simulink model "Scattering_based_Position_Position_discrete"  (R2020b)
settings: Solver=VariableStepAuto  StartTime=0.0  StopTime=10  RelTol=1e-3
values from neighbouring files (symbols this model uses):
  Amp = 1    [parameters_Position_Position.m]    (also in parameters_Position_Position_kalman.m)
  b = 1    [parameters_Position_Position.m]    (also in parameters_Position_Position_kalman.m)
  Be = 10    [parameters_Position_Position.m]    (also in parameters_Position_Position_kalman.m)
  Bh = 1.5    [parameters_Position_Position.m]    (also in parameters_Position_Position_kalman.m)
  Bm = 100    [parameters_Position_Position.m]    (also in parameters_Position_Position_kalman.m)
  Bs = 100    [parameters_Position_Position.m]    (also in parameters_Position_Position_kalman.m)
  delay = 1    [parameters_Position_Position.m]    (also in parameters_Position_Position_kalman.m)
  Dm = 0    [parameters_Position_Position.m]    (also in parameters_Position_Position_kalman.m)
  Ds = 0    [parameters_Position_Position.m]    (also in parameters_Position_Position_kalman.m)
  Fc = 0.5    [parameters_Position_Position.m]    (also in parameters_Position_Position_kalman.m)
  Fip = 100    [parameters_Position_Position.m]    (also in parameters_Position_Position_kalman.m)
  Ih = 5    [parameters_Position_Position.m]    (also in parameters_Position_Position_kalman.m)
  Je = 0    [parameters_Position_Position.m]    (also in parameters_Position_Position_kalman.m)
  Jh = 0    [parameters_Position_Position.m]    (also in parameters_Position_Position_kalman.m)
  Ke = 10    [parameters_Position_Position.m]    (also in parameters_Position_Position_kalman.m)
  Kh = 1    [parameters_Position_Position.m]    (also in parameters_Position_Position_kalman.m)
  Km = 50    [parameters_Position_Position.m]    (also in parameters_Position_Position_kalman.m)
  Ks = 80    [parameters_Position_Position.m]    (also in parameters_Position_Position_kalman.m)
  Mm = 0.5    [parameters_Position_Position.m]    (also in parameters_Position_Position_kalman.m)
  Ms = 2    [parameters_Position_Position.m]    (also in parameters_Position_Position_kalman.m)
  Ph = 5    [parameters_Position_Position.m]    (also in parameters_Position_Position_kalman.m)
  tau = 100000    [parameters_Position_Position.m]    (also in parameters_Position_Position_kalman.m)
  Ts = 0.001    [parameters_Position_Position.m]    (also in parameters_Position_Position_kalman.m)
undefined symbols (not defined in the file or in its folder): DiscIntNeverNeededParam
libraries: simulink x2
settings Model: Creator=anuj  LastModifiedBy=Edoardo

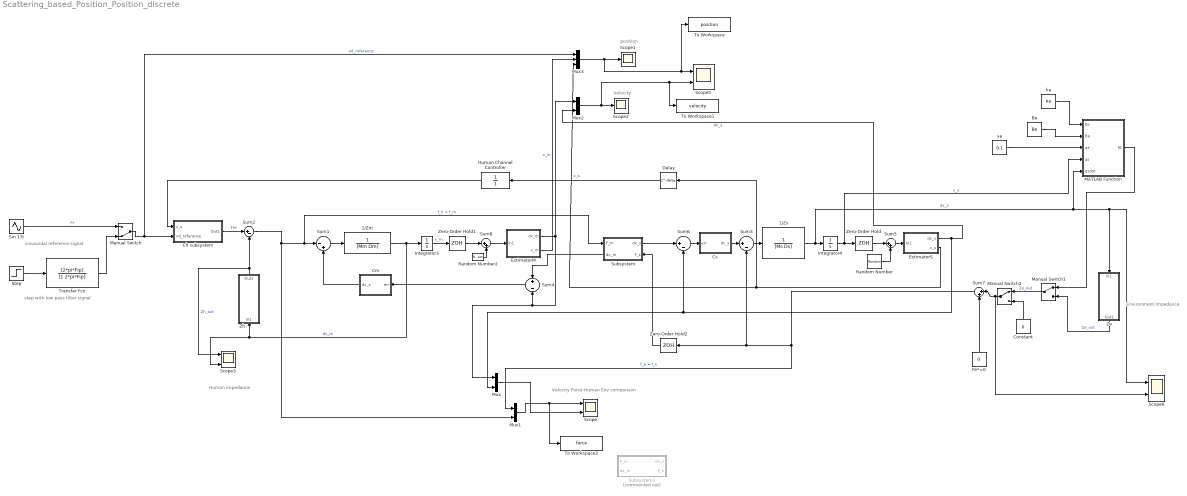
== system Scattering_based_Position_Position_discrete ==
  note: Velocity
  note: position
  note: Environment Impedance
  note: Human impedance
  note: Velocity Force Human Env comparison
  note: sinusoidal reference signal
  note: step with low pass filter signal
  1/Zm : TransferFcn  Denominator=[Mm Dm]
  1/Zs : TransferFcn  Denominator=[Ms Ds]
  Be : Constant  Value=Be
  Ch subsystem : Subsystem
  Cm : Subsystem
  Constant : Constant  Value=0
  Cs : Subsystem
  Delay : Delay  DelayLength=delay  SampleTime=Ts
  EstimatorM : Subsystem
  EstimatorS : Subsystem
  Fe*=0 : Constant  Value=0
  Human Channel Controller : TransferFcn  Denominator=[1]
  Integrator3 : Integrator
  Integrator4 : Integrator
  MATLAB Function : MATLAB Function  TreatAsAtomicUnit=on
  Manual Switch : ManualSwitch  CurrentSetting=0
  Manual Switch1 : ManualSwitch
  Manual Switch2 : ManualSwitch
  Mux : Mux  Inputs=2
  Mux1 : Mux  Inputs=2
  Mux2 : Mux  Inputs=2
  Mux3 : Mux  Inputs=3
  Random Number : RandomNumber  Variance=0  SampleTime=0.1
  Random Number2 : RandomNumber  Variance=0  SampleTime=0.1
  Scope{,3,5..6} (4 alike) : Scope  NumInputPorts=2
  Scope1 : Scope
  Scope2 : Scope
  Sin 17t : Sin  Amplitude=Amp  Frequency=2*pi*Fc  SampleTime=0
  Step : Step  After=Amp  SampleTime=0
  Subsystem : Subsystem
      settings: PortSchema="{\"entries\":[{\"content\":{\"sides\":[{\"content\":{\"connectorIds\":[\"In1\",\"Out2\"]},\"type\":\"ConnectorPlacement.EquallySpacedRectSide\",\"uuid\":\"a4d8a1e6-493d-445f-9b62-4880423e0f65\"},{\"content\":{\"connectorIds\":[\"Out1\",\"In2\"],\"side\":\"RIGHT\"},\"type\":\"ConnectorPlacement.EquallySpacedRectSide\",\"uuid\":\"3d032ce1-a127-47bd-8907-4bd2e1f875d6\"},{\"content\":{\"connectorIds\":[],\"side\":\"TOP\"},\"type\":\"ConnectorPlacement.EquallySpacedRectSide\",\"uuid\":\"51a1971f-6e89-4837-8aa9-c8a237b527d1\"},{\"content\":{\"connectorIds\":[],\"side\":\"HIDDEN\"},\"type\":\"ConnectorPlacement.EquallySpacedRectSide\",\"uuid\":\"2bd12734-fa67-440d-bc97-b4fe58bfa138\"}]},\"type\":\"ConnectorPlacement.EquallySpacedConnector\",\"uuid\":\"cc0f3456-b5e1-4f18-b500-07b4336c0d17\"}],\"packageUris\":[\"http://schema.mathworks.com/mf0/Connector/R2020b\"],\"version\":\"1.0\"}"
  Subsystem1 : Subsystem  Commented=on
      settings: PortSchema="{\"entries\":[{\"content\":{\"sides\":[{\"content\":{\"connectorIds\":[\"In1\",\"Out2\"]},\"type\":\"ConnectorPlacement.EquallySpacedRectSide\",\"uuid\":\"06c9fa59-43a1-4b94-81eb-aaec109dce8e\"},{\"content\":{\"connectorIds\":[\"Out1\",\"In2\"],\"side\":\"RIGHT\"},\"type\":\"ConnectorPlacement.EquallySpacedRectSide\",\"uuid\":\"3f5f1dc1-0465-4088-8d45-d4d0bf9b65eb\"},{\"content\":{\"connectorIds\":[],\"side\":\"TOP\"},\"type\":\"ConnectorPlacement.EquallySpacedRectSide\",\"uuid\":\"9f406951-78e1-44a4-92d9-8338b6137a61\"},{\"content\":{\"connectorIds\":[],\"side\":\"HIDDEN\"},\"type\":\"ConnectorPlacement.EquallySpacedRectSide\",\"uuid\":\"c520c54c-b8c0-41cc-b366-9b185ca7cd6e\"}]},\"type\":\"ConnectorPlacement.EquallySpacedConnector\",\"uuid\":\"d081af34-e020-4561-aa1f-800c2949a30c\"}],\"packageUris\":[\"http://schema.mathworks.com/mf0/Connector/R2020b\"],\"version\":\"1.0\"}"
  Sum1 : Sum  Inputs=|-+
  Sum2 : Sum  Inputs=|+-
  Sum3 : Sum  Inputs=|+-
  Sum4 : Sum  Inputs=+-
  Sum5 : Sum  Inputs=|++
  Sum6 : Sum  Inputs=|+-
  Sum7 : Sum  Inputs=|++
  Sum8 : Sum  Inputs=|++
  To Workspace : ToWorkspace  VariableName=position  SaveFormat=Timeseries  SampleTime=-1
  To Workspace1 : ToWorkspace  VariableName=velocity  SaveFormat=Timeseries  SampleTime=-1
  To Workspace2 : ToWorkspace  VariableName=force  SaveFormat=Timeseries  SampleTime=-1
  Transfer Fcn : TransferFcn  Numerator=[2*pi*Fip]  Denominator=[1 2*pi*Fip]
  Ze : Subsystem
  Zero-Order Hold : ZeroOrderHold  SampleTime=Ts
  Zero-Order Hold1 : ZeroOrderHold  SampleTime=Ts
  Zero-Order Hold2 : ZeroOrderHold  SampleTime=-1
  Zh : Subsystem
  ke : Constant  Value=Ke
  xe : Constant  Value=0.1
  wires:
  Mux/1 -> Scope/2
  Mux1/1 -> Scope/1, To Workspace2/1
  Sum2/1 -> Subsystem/1(F_m), Sum1/1, Mux1/2  "f_h = f_m"
  Sum1/1 -> 1/Zm/1
  Sum3/1 -> 1/Zs/1
  Fe*=0/1 -> Sum7/2
  Sum7/1 -> Mux1/1, Zero-Order Hold2/1, Sum3/2  "f_e = f_s"
  Ch subsystem/1(Out1) -> Sum2/1  "Fh*"
  Be/1 -> MATLAB Function/2(Be)
  xe/1 -> MATLAB Function/3(qe)
  ke/1 -> MATLAB Function/1(Ke)
  Transfer Fcn/1 -> Manual Switch/2
  Step/1 -> Transfer Fcn/1
  Human Channel Controller/1 -> Ch subsystem/1(x_s)
  Manual Switch/1 -> Mux3/1, Ch subsystem/2(xd_reference)  "xd_reference"
  Sin 17t/1 -> Manual Switch/1  "F*"
  MATLAB Function/1(fE) -> Manual Switch1/1
  Manual Switch1/1 -> Manual Switch2/1  "Ze_out"
  Zh/1(Out1) -> Sum2/2, Scope3/1  "Zh_out"
  Ze/1(Out1) -> Manual Switch1/2  "Ze_out"
  Mux2/1 -> Scope2/1, To Workspace1/1, Scope5/2
  Mux3/1 -> Scope1/1, To Workspace/1, Scope5/1
  Sum8/1 -> EstimatorM/1(In1)
  Random Number2/1 -> Sum8/2
  1/Zm/1 -> Integrator3/1, Zh/1(In1), Scope3/2  "dx_m"
  Zero-Order Hold1/1 -> Sum8/1
  Integrator3/1 -> Zero-Order Hold1/1  "x_m"
  EstimatorM/1(dx_m) -> Mux2/1, Sum4/2, Mux/1
  Sum5/1 -> EstimatorS/1(In1)
  Random Number/1 -> Sum5/2
  Zero-Order Hold/1 -> Sum5/1
  Integrator4/1 -> Zero-Order Hold/1, MATLAB Function/4(qs)  "x_s"
  EstimatorS/2(x_s) -> Delay/1, Mux3/3  "x_s"
  EstimatorS/1(dx_s) -> Mux/2, Sum6/2, Mux2/2  "dx_s"
  1/Zs/1 -> Ze/1(In1), Scope6/1, MATLAB Function/5(qsdot), Integrator4/1  "dx_s"
  EstimatorM/2(x_m) -> Mux3/2  "x_m"
  Zero-Order Hold2/1 -> Subsystem/2(F_s)
  Cs/1(dx_s) -> Sum3/1
  Subsystem/1(dx_s) -> Sum6/1
  Sum6/1 -> Cs/1(err)
  Manual Switch2/1 -> Scope6/2, Sum7/1
  Constant/1 -> Manual Switch2/2
  Subsystem/2(dx_m) -> Sum4/1
  Sum4/1 -> Cm/1(err)
  Cm/1(dx_s) -> Sum1/2
  Delay/1 -> Human Channel Controller/1

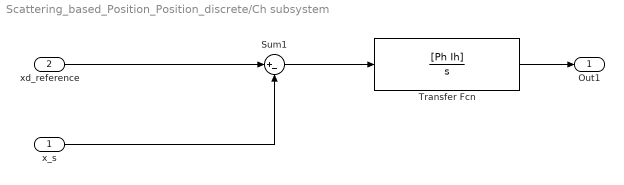
== system Scattering_based_Position_Position_discrete/Ch subsystem ==
  x_s : Inport
  xd_reference : Inport  Port=2
  Sum1 : Sum  Inputs=|+-
  Transfer Fcn : TransferFcn  Numerator=[Ph Ih]  Denominator=[1 0]
  Out1 : Outport
  wires:
  x_s/1 -> Sum1/2
  Sum1/1 -> Transfer Fcn/1
  xd_reference/1 -> Sum1/1
  Transfer Fcn/1 -> Out1/1

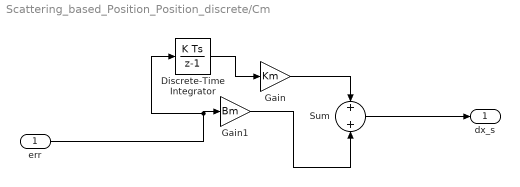
== system Scattering_based_Position_Position_discrete/Cm ==
  err : Inport
  Discrete-Time Integrator : DiscreteIntegrator  SampleTime=Ts  ICPrevOutput=DiscIntNeverNeededParam  ICPrevScaledInput=DiscIntNeverNeededParam
  Gain : Gain  Gain=Km
  Gain1 : Gain  Gain=Bm
  Sum : Sum
  dx_s : Outport
  wires:
  Gain1/1 -> Sum/2
  err/1 -> Discrete-Time Integrator/1, Gain1/1
  Discrete-Time Integrator/1 -> Gain/1
  Gain/1 -> Sum/1
  Sum/1 -> dx_s/1

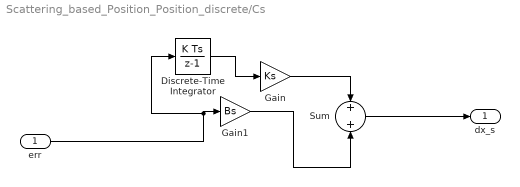
== system Scattering_based_Position_Position_discrete/Cs ==
  err : Inport
  Discrete-Time Integrator : DiscreteIntegrator  SampleTime=Ts  ICPrevOutput=DiscIntNeverNeededParam  ICPrevScaledInput=DiscIntNeverNeededParam
  Gain : Gain  Gain=Ks
  Gain1 : Gain  Gain=Bs
  Sum : Sum
  dx_s : Outport
  wires:
  Gain1/1 -> Sum/2
  err/1 -> Discrete-Time Integrator/1, Gain1/1
  Discrete-Time Integrator/1 -> Gain/1
  Gain/1 -> Sum/1
  Sum/1 -> dx_s/1

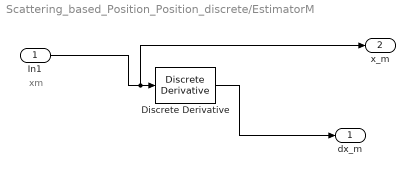
== system Scattering_based_Position_Position_discrete/EstimatorM ==
  note: xm
  In1 : Inport
  Discrete Derivative : simulink/Discrete/Discrete Derivative  gainval=1.0  ICPrevScaledInput=0.0  OutMin=[]  OutMax=[]  OutDataType=fixdt(1, 16)  OutScaling=2^-10  DoSatur=off
  dx_m : Outport
  x_m : Outport  Port=2
  wires:
  Discrete Derivative/1 -> dx_m/1
  In1/1 -> x_m/1, Discrete Derivative/1

== system Scattering_based_Position_Position_discrete/EstimatorS ==
  note: xs
  In1 : Inport
  Discrete Derivative : simulink/Discrete/Discrete Derivative  gainval=1.0  ICPrevScaledInput=0.0  OutMin=[]  OutMax=[]  OutDataType=fixdt(1, 16)  OutScaling=2^-10  DoSatur=off
  dx_s : Outport
  x_s : Outport  Port=2
  wires:
  In1/1 -> x_s/1, Discrete Derivative/1
  Discrete Derivative/1 -> dx_s/1

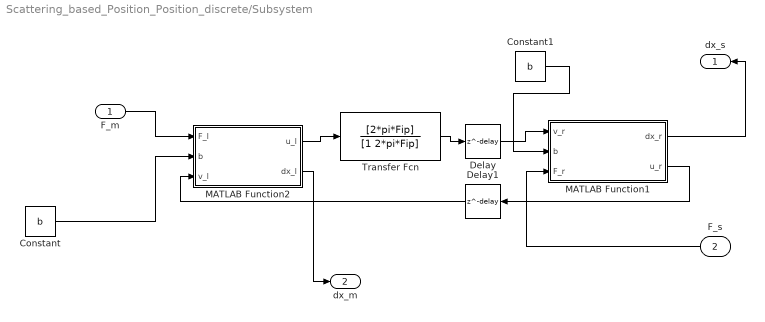
== system Scattering_based_Position_Position_discrete/Subsystem ==
  F_m : Inport
  F_s : Inport  Port=2
  Constant : Constant  Value=b
  Constant1 : Constant  Value=b
  Delay : Delay  DelayLength=delay  SampleTime=Ts
  Delay1 : Delay  DelayLength=delay  SampleTime=Ts
  MATLAB Function1 : MATLAB Function  TreatAsAtomicUnit=on
  MATLAB Function2 : MATLAB Function  TreatAsAtomicUnit=on
  Transfer Fcn : TransferFcn  Numerator=[2*pi*Fip]  Denominator=[1 2*pi*Fip]
  dx_s : Outport
  dx_m : Outport  Port=2
  wires:
  F_m/1 -> MATLAB Function2/1(F_l)
  MATLAB Function2/2(dx_l) -> dx_m/1
  MATLAB Function2/1(u_l) -> Transfer Fcn/1
  Delay/1 -> MATLAB Function1/1(v_r)
  Delay1/1 -> MATLAB Function2/3(v_l)
  MATLAB Function1/2(u_r) -> Delay1/1
  MATLAB Function1/1(dx_r) -> dx_s/1
  F_s/1 -> MATLAB Function1/3(F_r)
  Constant/1 -> MATLAB Function2/2(b)
  Constant1/1 -> MATLAB Function1/2(b)
  Transfer Fcn/1 -> Delay/1

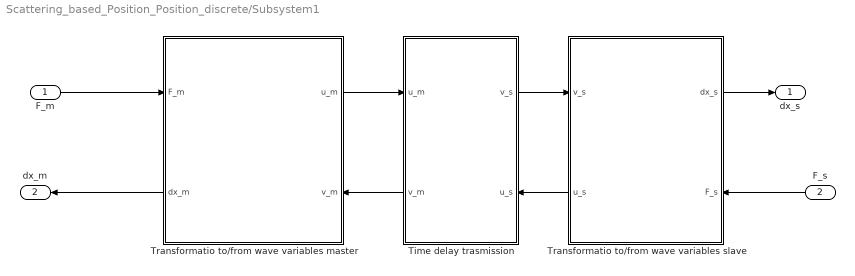
== system Scattering_based_Position_Position_discrete/Subsystem1 ==
  F_m : Inport
  F_s : Inport  Port=2
  Time delay trasmission : Subsystem
      settings: PortSchema="{\"entries\":[{\"content\":{\"sides\":[{\"content\":{\"connectorIds\":[\"In1\",\"Out2\"]},\"type\":\"ConnectorPlacement.EquallySpacedRectSide\",\"uuid\":\"c61cc498-c2d4-4974-8092-d1dd7246970f\"},{\"content\":{\"connectorIds\":[\"Out1\",\"In2\"],\"side\":\"RIGHT\"},\"type\":\"ConnectorPlacement.EquallySpacedRectSide\",\"uuid\":\"b3432fad-c145-4544-8ece-ee02518aa819\"},{\"content\":{\"connectorIds\":[],\"side\":\"TOP\"},\"type\":\"ConnectorPlacement.EquallySpacedRectSide\",\"uuid\":\"a4c87c21-faf5-4231-acac-6c0cf917f100\"},{\"content\":{\"connectorIds\":[],\"side\":\"BOTTOM\"},\"type\":\"ConnectorPlacement.EquallySpacedRectSide\",\"uuid\":\"b7041279-2e83-4165-9bf8-6e04fc95396e\"},{\"content\":{\"connectorIds\":[],\"side\":\"HIDDEN\"},\"type\":\"ConnectorPlacement.EquallySpacedRectSide\",\"uuid\":\"05f7a0d6-3baf-4f93-bf49-00ef202e853a\"}]},\"type\":\"ConnectorPlacement.EquallySpacedConnector\",\"uuid\":\"62683b5c-72e0-4cd5-964e-7729887f146f\"}],\"packageUris\":[\"http://schema.mathworks.com/mf0/Connector/R2020b\"],\"version\":\"1.0\"}"
  Transformatio to/from wave variables master : Subsystem
      settings: PortSchema="{\"entries\":[{\"content\":{\"sides\":[{\"content\":{\"connectorIds\":[\"In1\",\"Out2\"]},\"type\":\"ConnectorPlacement.EquallySpacedRectSide\",\"uuid\":\"c61cc498-c2d4-4974-8092-d1dd7246970f\"},{\"content\":{\"connectorIds\":[\"Out1\",\"In2\"],\"side\":\"RIGHT\"},\"type\":\"ConnectorPlacement.EquallySpacedRectSide\",\"uuid\":\"b3432fad-c145-4544-8ece-ee02518aa819\"},{\"content\":{\"connectorIds\":[],\"side\":\"TOP\"},\"type\":\"ConnectorPlacement.EquallySpacedRectSide\",\"uuid\":\"a4c87c21-faf5-4231-acac-6c0cf917f100\"},{\"content\":{\"connectorIds\":[],\"side\":\"BOTTOM\"},\"type\":\"ConnectorPlacement.EquallySpacedRectSide\",\"uuid\":\"b7041279-2e83-4165-9bf8-6e04fc95396e\"},{\"content\":{\"connectorIds\":[],\"side\":\"HIDDEN\"},\"type\":\"ConnectorPlacement.EquallySpacedRectSide\",\"uuid\":\"05f7a0d6-3baf-4f93-bf49-00ef202e853a\"}]},\"type\":\"ConnectorPlacement.EquallySpacedConnector\",\"uuid\":\"62683b5c-72e0-4cd5-964e-7729887f146f\"}],\"packageUris\":[\"http://schema.mathworks.com/mf0/Connector/R2020b\"],\"version\":\"1.0\"}"
  Transformatio to/from wave variables slave : Subsystem
      settings: PortSchema="{\"entries\":[{\"content\":{\"sides\":[{\"content\":{\"connectorIds\":[\"In1\",\"Out2\"]},\"type\":\"ConnectorPlacement.EquallySpacedRectSide\",\"uuid\":\"c61cc498-c2d4-4974-8092-d1dd7246970f\"},{\"content\":{\"connectorIds\":[\"Out1\",\"In2\"],\"side\":\"RIGHT\"},\"type\":\"ConnectorPlacement.EquallySpacedRectSide\",\"uuid\":\"b3432fad-c145-4544-8ece-ee02518aa819\"},{\"content\":{\"connectorIds\":[],\"side\":\"TOP\"},\"type\":\"ConnectorPlacement.EquallySpacedRectSide\",\"uuid\":\"a4c87c21-faf5-4231-acac-6c0cf917f100\"},{\"content\":{\"connectorIds\":[],\"side\":\"BOTTOM\"},\"type\":\"ConnectorPlacement.EquallySpacedRectSide\",\"uuid\":\"b7041279-2e83-4165-9bf8-6e04fc95396e\"},{\"content\":{\"connectorIds\":[],\"side\":\"HIDDEN\"},\"type\":\"ConnectorPlacement.EquallySpacedRectSide\",\"uuid\":\"05f7a0d6-3baf-4f93-bf49-00ef202e853a\"}]},\"type\":\"ConnectorPlacement.EquallySpacedConnector\",\"uuid\":\"62683b5c-72e0-4cd5-964e-7729887f146f\"}],\"packageUris\":[\"http://schema.mathworks.com/mf0/Connector/R2020b\"],\"version\":\"1.0\"}"
  dx_s : Outport
  dx_m : Outport  Port=2
  wires:
  Time delay trasmission/1(v_s) -> Transformatio to/from wave variables slave/1(v_s)
  Transformatio to/from wave variables master/1(u_m) -> Time delay trasmission/1(u_m)
  F_m/1 -> Transformatio to/from wave variables master/1(F_m)
  Transformatio to/from wave variables master/2(dx_m) -> dx_m/1
  F_s/1 -> Transformatio to/from wave variables slave/2(F_s)
  Transformatio to/from wave variables slave/1(dx_s) -> dx_s/1
  Time delay trasmission/2(v_m) -> Transformatio to/from wave variables master/2(v_m)
  Transformatio to/from wave variables slave/2(u_s) -> Time delay trasmission/2(u_s)

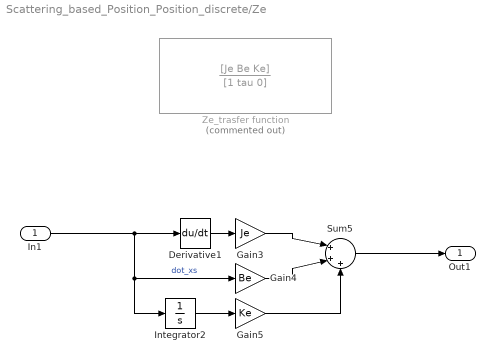
== system Scattering_based_Position_Position_discrete/Ze ==
  In1 : Inport
  Derivative1 : Derivative
  Gain3 : Gain  Gain=Je
  Gain4 : Gain  Gain=Be
  Gain5 : Gain  Gain=Ke
  Integrator2 : Integrator
  Sum5 : Sum  Inputs=|+++
  Ze_trasfer function : TransferFcn  Commented=on  Numerator=[Je Be Ke]  Denominator=[1 tau 0]
  Out1 : Outport
  wires:
  Gain4/1 -> Sum5/2
  Gain3/1 -> Sum5/1
  Gain5/1 -> Sum5/3
  Sum5/1 -> Out1/1
  Integrator2/1 -> Gain5/1
  In1/1 -> Integrator2/1, Gain4/1, Derivative1/1  "dot_xs"
  Derivative1/1 -> Gain3/1

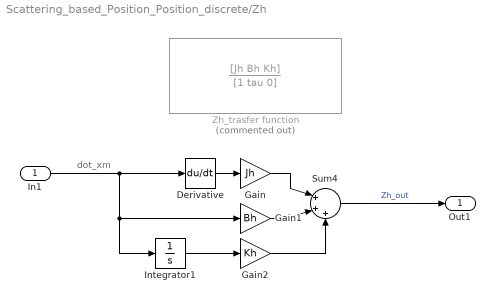
== system Scattering_based_Position_Position_discrete/Zh ==
  note: dot_xm
  In1 : Inport
  Derivative : Derivative
  Gain : Gain  Gain=Jh
  Gain1 : Gain  Gain=Bh
  Gain2 : Gain  Gain=Kh
  Integrator1 : Integrator
  Sum4 : Sum  Inputs=|+++
  Zh_trasfer function : TransferFcn  Commented=on  Numerator=[Jh Bh Kh]  Denominator=[1 tau 0]
  Out1 : Outport
  wires:
  Derivative/1 -> Gain/1
  Integrator1/1 -> Gain2/1
  Gain2/1 -> Sum4/3
  Gain1/1 -> Sum4/2
  Gain/1 -> Sum4/1
  Sum4/1 -> Out1/1  "Zh_out"
  In1/1 -> Gain1/1, Integrator1/1, Derivative/1

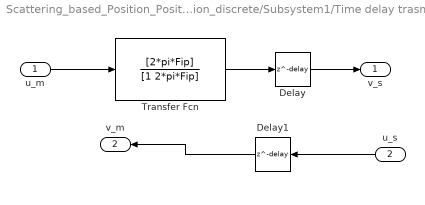
== system Scattering_based_Position_Position_discrete/Subsystem1/Time delay trasmission ==
  u_m : Inport
  u_s : Inport  Port=2
  Delay : Delay  DelayLength=delay  SampleTime=Ts
  Delay1 : Delay  DelayLength=delay  SampleTime=Ts
  Transfer Fcn : TransferFcn  Numerator=[2*pi*Fip]  Denominator=[1 2*pi*Fip]
  v_s : Outport
  v_m : Outport  Port=2
  wires:
  u_m/1 -> Transfer Fcn/1
  Transfer Fcn/1 -> Delay/1
  u_s/1 -> Delay1/1
  Delay/1 -> v_s/1
  Delay1/1 -> v_m/1

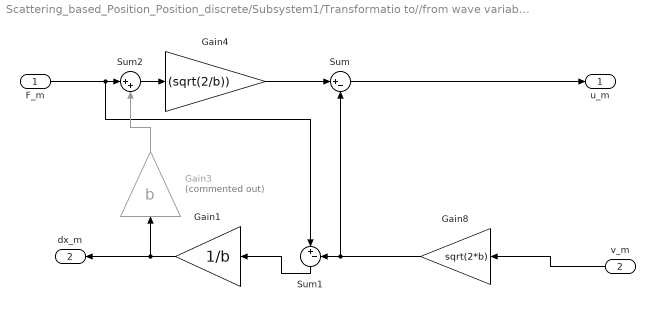
== system Scattering_based_Position_Position_discrete/Subsystem1/Transformatio to//from wave variables master ==
  F_m : Inport
  v_m : Inport  Port=2
  Gain1 : Gain  Gain=1/b
  Gain3 : Gain  Commented=on  Gain=b
  Gain4 : Gain  Gain=(sqrt(2/b))
  Gain8 : Gain  Gain=sqrt(2*b)
  Sum : Sum  Inputs=|+-
  Sum1 : Sum  Inputs=|+-
  Sum2 : Sum  Inputs=|++
  u_m : Outport
  dx_m : Outport  Port=2
  wires:
  Sum2/1 -> Gain4/1
  Sum/1 -> u_m/1
  v_m/1 -> Gain8/1
  Sum1/1 -> Gain1/1
  F_m/1 -> Sum1/1, Sum2/1
  Gain3/1 -> Sum2/2
  Gain1/1 -> Gain3/1, dx_m/1
  Gain4/1 -> Sum/1
  Gain8/1 -> Sum/2, Sum1/2

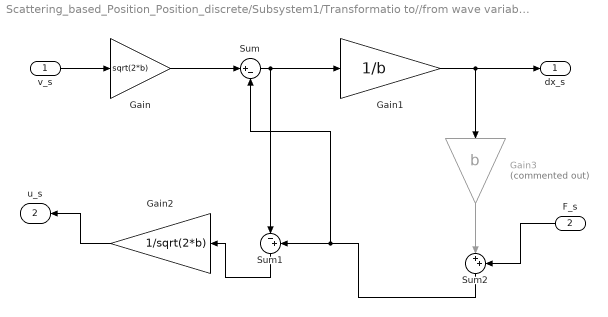
== system Scattering_based_Position_Position_discrete/Subsystem1/Transformatio to//from wave variables slave ==
  v_s : Inport
  F_s : Inport  Port=2
  Gain : Gain  Gain=sqrt(2*b)
  Gain1 : Gain  Gain=1/b
  Gain2 : Gain  Gain=1/sqrt(2*b)
  Gain3 : Gain  Commented=on  Gain=b
  Sum : Sum  Inputs=|+-
  Sum1 : Sum  Inputs=|-+
  Sum2 : Sum  Inputs=|++
  dx_s : Outport
  u_s : Outport  Port=2
  wires:
  Gain1/1 -> Gain3/1, dx_s/1
  Gain/1 -> Sum/1
  Sum2/1 -> Sum/2, Sum1/2
  v_s/1 -> Gain/1
  Sum1/1 -> Gain2/1
  Sum/1 -> Gain1/1, Sum1/1
  Gain2/1 -> u_s/1
  F_s/1 -> Sum2/2
  Gain3/1 -> Sum2/1

== matlab function Scattering_based_Position_Position_discrete/Subsystem/MATLAB Function2 ==
  data: F_l input; b input; u_l output; v_l input; dx_l output
function [u_l, dx_l] = left(F_l, b, v_l)

u_l = sqrt(2/b)*F_l - v_l;
dx_l = 1/b*(F_l - sqrt(2*b)*v_l);

== matlab function Scattering_based_Position_Position_discrete/MATLAB Function ==
  data: Ke input; fE output; Be input; qe input; qs input; qsdot input
function fE = environment(Ke, Be, qe, qs, qsdot)
    if qs > qe
        fE = Ke * (qs - qe) + Be * qsdot;
    else
        fE = 0;
    end
end

== matlab function Scattering_based_Position_Position_discrete/Subsystem/MATLAB Function1 ==
  data: v_r input; b input; dx_r output; F_r input; u_r output
function [dx_r, u_r] = right(v_r, b, F_r)

u_r  = sqrt(2/b)*F_r - v_r;
dx_r = -(1/b)*(F_r - sqrt(2*b)*v_r);
